simulink model "TheStepResponseCurveBeforeAndAfterCorrection"  (Simulink 8.9)
settings: Solver=VariableStepAuto  StartTime=0.0  StopTime=10.0  RelTol=1e-3
settings Model: Creator=xiang  LastModifiedBy=xiang
settings DataIOCC: LimitDataPoints=off  SaveFormat=Dataset  SignalLoggingSaveFormat=Dataset
settings OptimizationCC: LifeSpan=auto
settings DebuggingCC: UnderspecifiedInitializationDetection=Simplified  MergeDetectMultiDrivingBlocksExec=error  FcnCallInpInsideContextMsg=error  StateNameClashWarn=none  SFUnexpectedBacktrackingDiag=error  SFNoUnconditionalDefaultTransitionDiag=error  SFExecutionAtInitializationDiag=warning
settings HardwareCC: ProdBitPerPointer=64  ProdBitPerSizeT=64  ProdBitPerPtrDiffT=64  ProdLargestAtomicFloat=Float  ProdIntDivRoundTo=Zero  ProdEndianess=LittleEndian  ProdWordSize=64  ProdHWDeviceType=Intel->x86-64 (Windows64)
settings ModelReferenceCC: PropagateSignalLabelsOutOfModel=on
settings GRTTargetCC: TargetLangStandard=C99 (ISO)  GeneratePreprocessorConditionals=Use local settings  CombineOutputUpdateFcns=on  GRTInterface=off
settings ConfigComp: CovMetricSettings=dwe  CovHtmlReporting=off  CovSaveCumulativeToWorkspaceVar=off  CovSaveSingleToWorkspaceVar=off  CovExternalEMLEnable=on

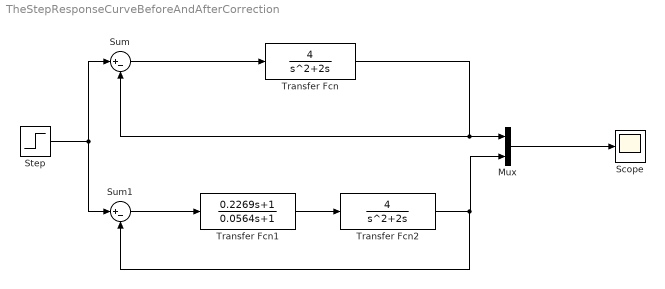
== system TheStepResponseCurveBeforeAndAfterCorrection ==
  Mux : Mux  Inputs=2
  Scope : Scope
  Step : Step  SampleTime=0
  Sum : Sum  Inputs=|+-
  Sum1 : Sum  Inputs=|+-
  Transfer Fcn : TransferFcn  Numerator=[4]  Denominator=[1 2 0]
  Transfer Fcn1 : TransferFcn  Numerator=[0.2269 1]  Denominator=[0.0564 1]
  Transfer Fcn2 : TransferFcn  Numerator=[4]  Denominator=[1 2 0]
  wires:
  Mux/1 -> Scope/1
  Transfer Fcn/1 -> Sum/2, Mux/1
  Transfer Fcn2/1 -> Sum1/2, Mux/2
  Transfer Fcn1/1 -> Transfer Fcn2/1
  Sum1/1 -> Transfer Fcn1/1
  Step/1 -> Sum/1, Sum1/1
  Sum/1 -> Transfer Fcn/1
